simulink model "simuElectro"  (R2024b)
settings: Solver=VariableStepAuto  StartTime=0.0  StopTime=10.0  RelTol=1e-3
values from neighbouring files (symbols this model uses):
  b = 0.0012    [motorDC_ode45.m]
  Jm = 0.001    [motorDC_ode45.m]
  Ke = 0.01    [motorDC_ode45.m]
  Kt = 0.01    [motorDC_ode45.m]
  La = 0.023    [motorDC_ode45.m]
  Ra = 2    [motorDC_ode45.m]
settings Model: Creator=USER
settings RTWCC: GPUComputeCapability=3.5

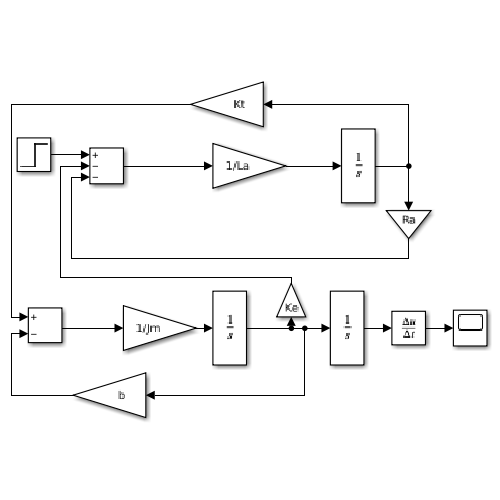
[thumbnail: Simulink's stored preview of the top-level diagram]
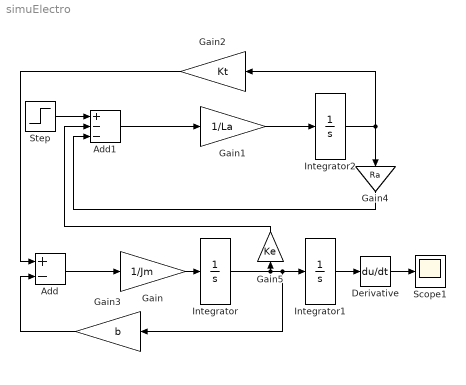
== system simuElectro ==
  Add : Sum  Inputs=+-
  Add1 : Sum  Inputs=+--
  Derivative : Derivative
  Gain : Gain  Gain=1/Jm
  Gain1 : Gain  Gain=1/La
  Gain2 : Gain  Gain=Kt
  Gain3 : Gain  Gain=b
  Gain4 : Gain  Gain=Ra
  Gain5 : Gain  Gain=Ke
  Integrator : Integrator
  Integrator1 : Integrator
  Integrator2 : Integrator
  Scope1 : Scope
  Step : Step  Time=0  After=5  SampleTime=0
  wires:
  Integrator/1 -> Gain3/1, Integrator1/1, Gain5/1
  Gain/1 -> Integrator/1
  Add/1 -> Gain/1
  Gain1/1 -> Integrator2/1
  Add1/1 -> Gain1/1
  Integrator1/1 -> Derivative/1
  Integrator2/1 -> Gain2/1, Gain4/1
  Gain2/1 -> Add/1
  Gain3/1 -> Add/2
  Step/1 -> Add1/1
  Derivative/1 -> Scope1/1
  Gain5/1 -> Add1/2
  Gain4/1 -> Add1/3
